simulink model "Q2C"  (R2021b)
settings: Solver=FixedStepAuto  StartTime=0.0  StopTime=1  FixedStep=100e-6  RelTol=1e-3
settings Model: Creator=yyx  LastModifiedBy=Divin

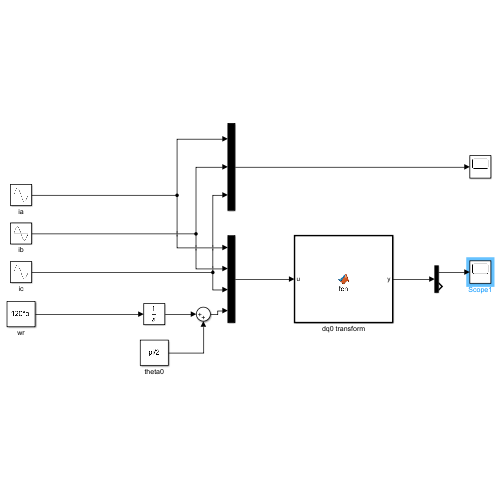
[thumbnail: Simulink's stored preview of the top-level diagram]
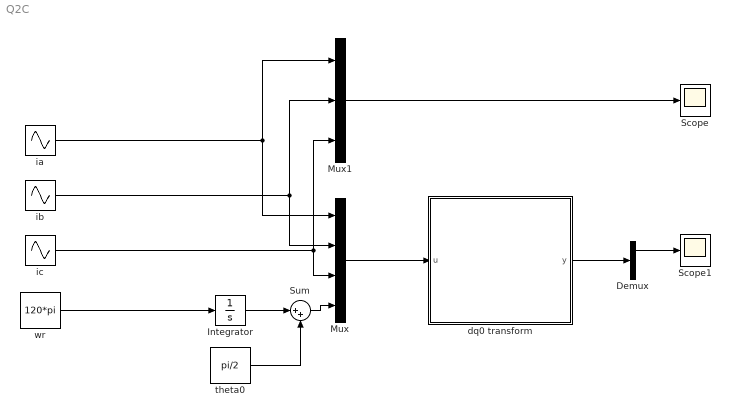
== system Q2C ==
  Demux : Demux  Outputs=2
  Integrator : Integrator
  Mux : Mux
  Mux1 : Mux  Inputs=3
  Scope : Scope
  Scope1 : Scope
  Sum : Sum  Inputs=|++
  dq0 transform : MATLAB Function  TreatAsAtomicUnit=on
  ia : Sin  Frequency=2*pi*60  SampleTime=0
  ib : Sin  Frequency=2*pi*60  Phase=-2*pi/3  SampleTime=0
  ic : Sin  Frequency=2*pi*60  Phase=2*pi/3  SampleTime=0
  theta0 : Constant  Value=pi/2
  wr : Constant  Value=120*pi
  wires:
  wr/1 -> Integrator/1
  Mux/1 -> dq0 transform/1(u)
  ia/1 -> Mux1/1, Mux/1
  ib/1 -> Mux/2, Mux1/2
  ic/1 -> Mux/3, Mux1/3
  dq0 transform/1(y) -> Demux/1
  Integrator/1 -> Sum/1
  theta0/1 -> Sum/2
  Sum/1 -> Mux/4
  Mux1/1 -> Scope/1
  Demux/1 -> Scope1/1

== matlab function Q2C/dq0 transform ==
  data: u input; y output
function y = fcn(u)


id = (2/3)*(cos(u(4))*u(1)+cos(u(4)-2*pi/3)*u(2)+cos(u(4)+2*pi/3)*u(3));
iq = (2/3)*(-sin(u(4))*u(1)-sin(u(4)-2*pi/3)*u(2)-sin(u(4)+2*pi/3)*u(3));
i0 = (1/3)*(u(1)+u(2)+u(3));
y = [id,iq,i0];
